simulink model "pushbullet_task"  (Simulink 3.00)
undefined symbols (not defined in the file): application, json
libraries: stringlib x7, mathlib x3, speclib x1

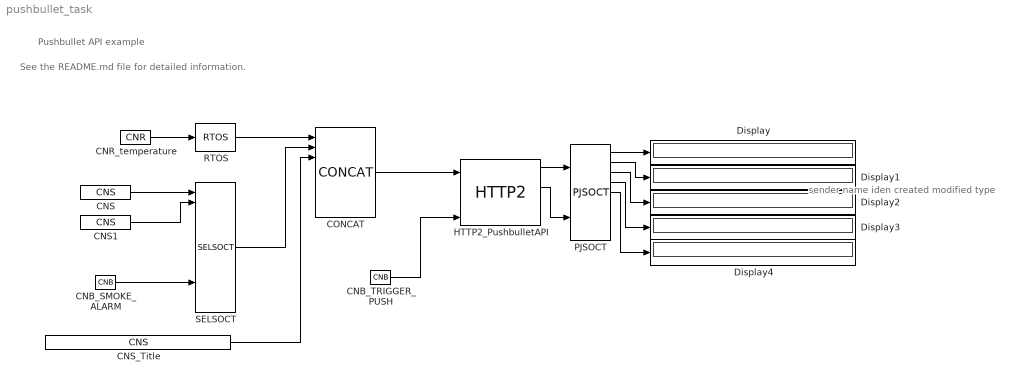
== system pushbullet_task ==
  note: See the README.md file for detailed information.
  note: Pushbullet API example
  note: sender name
      |
      | iden
      |
      | created
      |
      | modified
      |
      | type
  CNB_SMOKE_ALARM : mathlib/CNB  YCN=on
  CNB_TRIGGER_PUSH : mathlib/CNB  YCN=off
  CNR_temperature : mathlib/CNR  ycn=21.7
  CNS : stringlib/CNS  scv=inactive  nmax=0
  CNS1 : stringlib/CNS  scv=active  nmax=0
  CNS_Title : stringlib/CNS  scv=Message from REX  nmax=0
  CONCAT : stringlib/CONCAT  ptrn="{\"body\":\"Hi there, this is a message from REX. Temperature is %1 and the smoke sensor is %2. Have a nice day!\",\"title\":\"%3\",\"type\":\"note\"}"  nmax=0
  Display{,1..4} (5 alike) : Display
      settings: Format=Best fit
  HTTP2_PushbulletAPI : speclib/HTTP2  url=https://api.pushbullet.com/v2/pushes  method=2: POST  user=YourAccessToken  VERIFY=off  postmime=application/json  acceptmime=application/json  timeout=5  BLOCKING=off  nmax=0  postmax=256  datamax=1024
  PJSOCT : stringlib/PJSOCT  name1=sender_name  name2=iden  name3=created  name4=modified  name5=type  nmax=0
  RTOS : stringlib/RTOS  prec=5  mode=1: best fit
  SELSOCT : stringlib/SELSOCT  BINF=on  nmax=0
  wires:
  CNB_SMOKE_ALARM/1 -> SELSOCT/10
  CNB_TRIGGER_PUSH/1 -> HTTP2_PushbulletAPI/4
  CNR_temperature/1 -> RTOS/1
  CNS/1 -> SELSOCT/1
  CNS1/1 -> SELSOCT/2
  CNS_Title/1 -> CONCAT/3
  CONCAT/1 -> HTTP2_PushbulletAPI/1
  HTTP2_PushbulletAPI/1 -> PJSOCT/1
  HTTP2_PushbulletAPI/3 -> PJSOCT/2
  PJSOCT/1 -> Display/1
  PJSOCT/2 -> Display1/1
  PJSOCT/3 -> Display2/1
  PJSOCT/4 -> Display3/1
  PJSOCT/5 -> Display4/1
  RTOS/1 -> CONCAT/1
  SELSOCT/1 -> CONCAT/2
